simulink model "structuri_avansate"  (R2024a)
settings: Solver=VariableStepAuto  StartTime=0.0  StopTime=1000  RelTol=1e-3
values from neighbouring files (symbols this model uses):
  C = 9    [Proiect.m]
  h0 = 16.78    [Proiect.m]
  h1 = 19.66    [Proiect.m]
  k = 0.035    [Proiect.m]
  k11 = k2*k2+4*(k-k3)*k1    (= 0.0890826)    [Proiect.m]
  k12 = 8*(k-k3)    (= 0.2848)    [Proiect.m]
  k13 = 2*(k-k3)    (= 0.0712)    [Proiect.m]
  k2 = -0.015    [Proiect.m]
  kcompensare = (delta_h/(q1-q0))/(delta_h/delta_ua)    (= 0.16393442623)    [Proiect.m]
  kp = (delta_h/3)/delta_ua    (= 1.92)    [Proiect.m]
  q0 = 37.07    [Proiect.m]
undefined symbols (not defined in the file or in its folder): ki, ki1, ki2, kp1, kp2
libraries: slpidlib x6
(part 1 of 2)
settings Model: Creator=cernu  LastModifiedBy=cernu

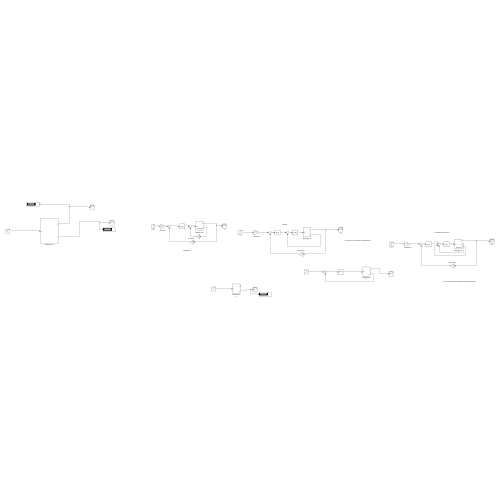
[thumbnail: Simulink's stored preview of the top-level diagram]
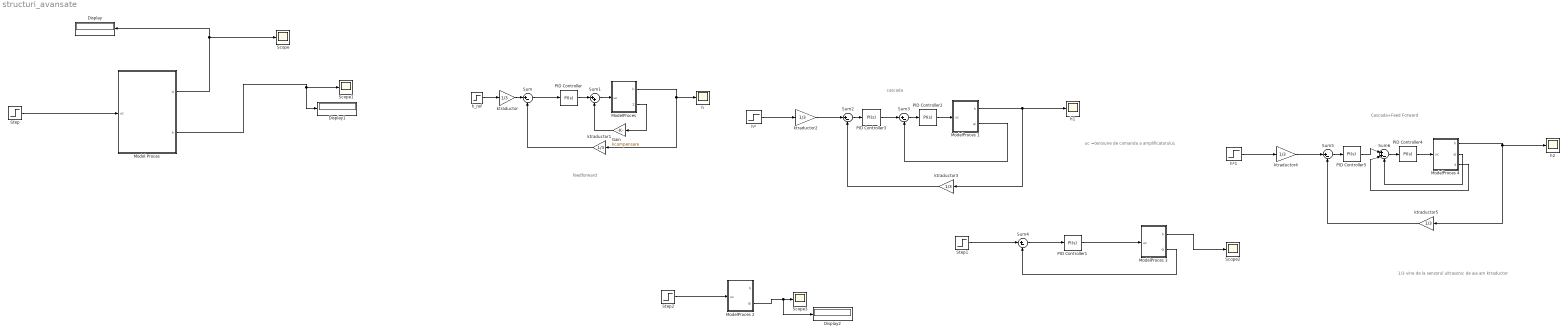
== system structuri_avansate ==
  note: 1/3 vine de la senzorul ultrasonic de aia am ktraductor
  note: Cascada+Feed Forward
  note: uc =tensiune de comanda a amplificatorului;
  note: cascada
  note: feedforward
  Display : Display
  Display1 : Display
  Display2 : Display
  Gain : Gain  Gain=kcompensare
  Model Proces : Subsystem
  "ModelProces " : Subsystem
  ModelProces 1 : Subsystem
  ModelProces 2 : Subsystem
  ModelProces 3 : Subsystem
  ModelProces 4 : Subsystem
  PID Controller : slpidlib/PID Controller  Controller=PI  Form=Parallel  TimeDomain=Continuous-time  UseExternalTs=off  SampleTime=-1  IntegratorMethod=Forward Euler  FilterMethod=Forward Euler  ControllerParametersSource=internal  P=kp  I=ki  UseKiTs=off  D=0  UseExternalDerivativeSource=off  N=100  UseFilter=on  TunerSelectOption=Transfer Function Based (PID Tuner App)  InitialConditionSource=internal  InitialConditionForIntegrator=6.7  InitialConditionForFilter=0  DifferentiatorICPrevScaledInput=0  ExternalReset=none  TrackingMode=off  Kt=1  LimitOutput=off  SatLimitsSource=internal  UpperSaturationLimit=inf  LowerSaturationLimit=-inf  LinearizeAsGain=on  AntiWindupMode=none  Kb=1  LimitIntegrator=off  UpperIntegratorSaturationLimit=inf  LowerIntegratorSaturationLimit=-inf  POutMin=[]  POutMax=[]  IOutMin=[]  IOutMax=[]  DOutMin=[]  DOutMax=[]  NOutMin=[]  NOutMax=[]  SumOutMin=[]  SumOutMax=[]  SaturationOutMin=[]  SaturationOutMax=[]  PParamMin=[]  PParamMax=[]  IParamMin=[]  IParamMax=[]  DParamMin=[]  DParamMax=[]  NParamMin=[]  NParamMax=[]  KbParamMin=[]  KbParamMax=[]  KtParamMin=[]  KtParamMax=[]  KbOutMin=[]  KbOutMax=[]  KtOutMin=[]  KtOutMax=[]  IntegratorOutMin=[]  IntegratorOutMax=[]  FilterOutMin=[]  FilterOutMax=[]  SumI1OutMin=[]  SumI1OutMax=[]  SumI2OutMin=[]  SumI2OutMax=[]  SumI3OutMin=[]  SumI3OutMax=[]  SumI4OutMin=[]  SumI4OutMax=[]  SumDOutMin=[]  SumDOutMax=[]  DifferentiatorOutMin=[]  DifferentiatorOutMax=[]  FilterDiffOutCoefMin=[]  FilterDiffOutCoefMax=[]  ReciprocalOutMin=[]  ReciprocalOutMax=[]  SumDenOutMin=[]  SumDenOutMax=[]  SumNumOutMin=[]  SumNumOutMax=[]  DivideOutMin=[]  DivideOutMax=[]  UdiffTsProdOutMin=[]  UdiffTsProdOutMax=[]  NTsProdOutMin=[]  NTsProdOutMax=[]  UintegralTsProdOutMin=[]  UintegralTsProdOutMax=[]  UngainTsProdOutMin=[]  UngainTsProdOutMax=[]  ClampingZeroOutDataTypeStr=Inherit: Inherit via back propagation  ClampingZeroOutMin=[]  ClampingZeroOutMax=[]  FilterDenConstantOutDataTypeStr=Inherit: Inherit via back propagation  FilterDenConstantOutMin=[]  FilterDenConstantOutMax=[]  PCopyOutDataTypeStr=Inherit: Inherit via back propagation  PCopyOutMin=[]  PCopyOutMax=[]  NCopyOutDataTypeStr=Inherit: Inherit via back propagation  NCopyOutMin=[]  NCopyOutMax=[]  IntegratorContinuousStateAttributes=''  IntegratorStateMustResolveToSignalObject=off  IntegratorRTWStateStorageClass=Auto  FilterContinuousStateAttributes=''  FilterStateMustResolveToSignalObject=off  FilterRTWStateStorageClass=Auto  ParallelPVariant=InternalParameters  IdealPVariant=Disabled  IVariant=InternalParameters  DVariant=Disabled  IntegratorVariant=Continuous  SatVariant=Disabled  AWVariant=Passthrough  PCopyVariant=Disabled  TRVariant=Disabled  FdbkBlocksVariant=Forward  IdealPFdbkVariant=Disabled  SatFdbkVariant=Disabled  DerivativeFilterVariant=Disabled  NVariant=Disabled  NCopyVariant=Disabled_SignalSpec  FilterICVariant=Disabled  IntegratorICVariant=InternalICs  ExternalResetVariant=Disabled  TRSumVariant=Passthrough  SumFdbkVariant=Disabled  SumVariant=Sum_PI  TsampFilterVariant=InternalTs  TsampNgainVariant=Passthrough  TsampIntegralVariant=Disabled_SignalSpec  ExternalSaturationOutDataTypeStr=Inherit: Same as second input  DerivativeSourceVariant=Disabled
  PID Controller1 : slpidlib/PID Controller  Controller=PI  Form=Parallel  TimeDomain=Continuous-time  UseExternalTs=off  SampleTime=-1  IntegratorMethod=Forward Euler  FilterMethod=Forward Euler  ControllerParametersSource=internal  P=kp1  I=ki1  UseKiTs=off  D=0  UseExternalDerivativeSource=off  N=100  UseFilter=on  TunerSelectOption=Transfer Function Based (PID Tuner App)  InitialConditionSource=internal  InitialConditionForIntegrator=6.7  InitialConditionForFilter=0  DifferentiatorICPrevScaledInput=0  ExternalReset=none  TrackingMode=off  Kt=1  LimitOutput=off  SatLimitsSource=internal  UpperSaturationLimit=inf  LowerSaturationLimit=-inf  LinearizeAsGain=on  AntiWindupMode=none  Kb=1  LimitIntegrator=off  UpperIntegratorSaturationLimit=inf  LowerIntegratorSaturationLimit=-inf  POutMin=[]  POutMax=[]  IOutMin=[]  IOutMax=[]  DOutMin=[]  DOutMax=[]  NOutMin=[]  NOutMax=[]  SumOutMin=[]  SumOutMax=[]  SaturationOutMin=[]  SaturationOutMax=[]  PParamMin=[]  PParamMax=[]  IParamMin=[]  IParamMax=[]  DParamMin=[]  DParamMax=[]  NParamMin=[]  NParamMax=[]  KbParamMin=[]  KbParamMax=[]  KtParamMin=[]  KtParamMax=[]  KbOutMin=[]  KbOutMax=[]  KtOutMin=[]  KtOutMax=[]  IntegratorOutMin=[]  IntegratorOutMax=[]  FilterOutMin=[]  FilterOutMax=[]  SumI1OutMin=[]  SumI1OutMax=[]  SumI2OutMin=[]  SumI2OutMax=[]  SumI3OutMin=[]  SumI3OutMax=[]  SumI4OutMin=[]  SumI4OutMax=[]  SumDOutMin=[]  SumDOutMax=[]  DifferentiatorOutMin=[]  DifferentiatorOutMax=[]  FilterDiffOutCoefMin=[]  FilterDiffOutCoefMax=[]  ReciprocalOutMin=[]  ReciprocalOutMax=[]  SumDenOutMin=[]  SumDenOutMax=[]  SumNumOutMin=[]  SumNumOutMax=[]  DivideOutMin=[]  DivideOutMax=[]  UdiffTsProdOutMin=[]  UdiffTsProdOutMax=[]  NTsProdOutMin=[]  NTsProdOutMax=[]  UintegralTsProdOutMin=[]  UintegralTsProdOutMax=[]  UngainTsProdOutMin=[]  UngainTsProdOutMax=[]  ClampingZeroOutDataTypeStr=Inherit: Inherit via back propagation  ClampingZeroOutMin=[]  ClampingZeroOutMax=[]  FilterDenConstantOutDataTypeStr=Inherit: Inherit via back propagation  FilterDenConstantOutMin=[]  FilterDenConstantOutMax=[]  PCopyOutDataTypeStr=Inherit: Inherit via back propagation  PCopyOutMin=[]  PCopyOutMax=[]  NCopyOutDataTypeStr=Inherit: Inherit via back propagation  NCopyOutMin=[]  NCopyOutMax=[]  IntegratorContinuousStateAttributes=''  IntegratorStateMustResolveToSignalObject=off  IntegratorRTWStateStorageClass=Auto  FilterContinuousStateAttributes=''  FilterStateMustResolveToSignalObject=off  FilterRTWStateStorageClass=Auto  ParallelPVariant=InternalParameters  IdealPVariant=Disabled  IVariant=InternalParameters  DVariant=Disabled  IntegratorVariant=Continuous  SatVariant=Disabled  AWVariant=Passthrough  PCopyVariant=Disabled  TRVariant=Disabled  FdbkBlocksVariant=Forward  IdealPFdbkVariant=Disabled  SatFdbkVariant=Disabled  DerivativeFilterVariant=Disabled  NVariant=Disabled  NCopyVariant=Disabled_SignalSpec  FilterICVariant=Disabled  IntegratorICVariant=InternalICs  ExternalResetVariant=Disabled  TRSumVariant=Passthrough  SumFdbkVariant=Disabled  SumVariant=Sum_PI  TsampFilterVariant=InternalTs  TsampNgainVariant=Passthrough  TsampIntegralVariant=Disabled_SignalSpec  ExternalSaturationOutDataTypeStr=Inherit: Same as second input  DerivativeSourceVariant=Disabled
  PID Controller2 : slpidlib/PID Controller  Controller=PI  Form=Parallel  TimeDomain=Continuous-time  UseExternalTs=off  SampleTime=-1  IntegratorMethod=Forward Euler  FilterMethod=Forward Euler  ControllerParametersSource=internal  P=kp1  I=ki1  UseKiTs=off  D=0  UseExternalDerivativeSource=off  N=100  UseFilter=on  TunerSelectOption=Transfer Function Based (PID Tuner App)  InitialConditionSource=internal  InitialConditionForIntegrator=6.7  InitialConditionForFilter=0  DifferentiatorICPrevScaledInput=0  ExternalReset=none  TrackingMode=off  Kt=1  LimitOutput=off  SatLimitsSource=internal  UpperSaturationLimit=inf  LowerSaturationLimit=-inf  LinearizeAsGain=on  AntiWindupMode=none  Kb=1  LimitIntegrator=off  UpperIntegratorSaturationLimit=inf  LowerIntegratorSaturationLimit=-inf  POutMin=[]  POutMax=[]  IOutMin=[]  IOutMax=[]  DOutMin=[]  DOutMax=[]  NOutMin=[]  NOutMax=[]  SumOutMin=[]  SumOutMax=[]  SaturationOutMin=[]  SaturationOutMax=[]  PParamMin=[]  PParamMax=[]  IParamMin=[]  IParamMax=[]  DParamMin=[]  DParamMax=[]  NParamMin=[]  NParamMax=[]  KbParamMin=[]  KbParamMax=[]  KtParamMin=[]  KtParamMax=[]  KbOutMin=[]  KbOutMax=[]  KtOutMin=[]  KtOutMax=[]  IntegratorOutMin=[]  IntegratorOutMax=[]  FilterOutMin=[]  FilterOutMax=[]  SumI1OutMin=[]  SumI1OutMax=[]  SumI2OutMin=[]  SumI2OutMax=[]  SumI3OutMin=[]  SumI3OutMax=[]  SumI4OutMin=[]  SumI4OutMax=[]  SumDOutMin=[]  SumDOutMax=[]  DifferentiatorOutMin=[]  DifferentiatorOutMax=[]  FilterDiffOutCoefMin=[]  FilterDiffOutCoefMax=[]  ReciprocalOutMin=[]  ReciprocalOutMax=[]  SumDenOutMin=[]  SumDenOutMax=[]  SumNumOutMin=[]  SumNumOutMax=[]  DivideOutMin=[]  DivideOutMax=[]  UdiffTsProdOutMin=[]  UdiffTsProdOutMax=[]  NTsProdOutMin=[]  NTsProdOutMax=[]  UintegralTsProdOutMin=[]  UintegralTsProdOutMax=[]  UngainTsProdOutMin=[]  UngainTsProdOutMax=[]  ClampingZeroOutDataTypeStr=Inherit: Inherit via back propagation  ClampingZeroOutMin=[]  ClampingZeroOutMax=[]  FilterDenConstantOutDataTypeStr=Inherit: Inherit via back propagation  FilterDenConstantOutMin=[]  FilterDenConstantOutMax=[]  PCopyOutDataTypeStr=Inherit: Inherit via back propagation  PCopyOutMin=[]  PCopyOutMax=[]  NCopyOutDataTypeStr=Inherit: Inherit via back propagation  NCopyOutMin=[]  NCopyOutMax=[]  IntegratorContinuousStateAttributes=''  IntegratorStateMustResolveToSignalObject=off  IntegratorRTWStateStorageClass=Auto  FilterContinuousStateAttributes=''  FilterStateMustResolveToSignalObject=off  FilterRTWStateStorageClass=Auto  ParallelPVariant=InternalParameters  IdealPVariant=Disabled  IVariant=InternalParameters  DVariant=Disabled  IntegratorVariant=Continuous  SatVariant=Disabled  AWVariant=Passthrough  PCopyVariant=Disabled  TRVariant=Disabled  FdbkBlocksVariant=Forward  IdealPFdbkVariant=Disabled  SatFdbkVariant=Disabled  DerivativeFilterVariant=Disabled  NVariant=Disabled  NCopyVariant=Disabled_SignalSpec  FilterICVariant=Disabled  IntegratorICVariant=InternalICs  ExternalResetVariant=Disabled  TRSumVariant=Passthrough  SumFdbkVariant=Disabled  SumVariant=Sum_PI  TsampFilterVariant=InternalTs  TsampNgainVariant=Passthrough  TsampIntegralVariant=Disabled_SignalSpec  ExternalSaturationOutDataTypeStr=Inherit: Same as second input  DerivativeSourceVariant=Disabled
  PID Controller3 : slpidlib/PID Controller  Controller=PI  Form=Parallel  TimeDomain=Continuous-time  UseExternalTs=off  SampleTime=-1  IntegratorMethod=Forward Euler  FilterMethod=Forward Euler  ControllerParametersSource=internal  P=kp2  I=ki2  UseKiTs=off  D=0  UseExternalDerivativeSource=off  N=100  UseFilter=on  TunerSelectOption=Transfer Function Based (PID Tuner App)  InitialConditionSource=internal  InitialConditionForIntegrator=q0  InitialConditionForFilter=0  DifferentiatorICPrevScaledInput=0  ExternalReset=none  TrackingMode=off  Kt=1  LimitOutput=off  SatLimitsSource=internal  UpperSaturationLimit=inf  LowerSaturationLimit=-inf  LinearizeAsGain=on  AntiWindupMode=none  Kb=1  LimitIntegrator=off  UpperIntegratorSaturationLimit=inf  LowerIntegratorSaturationLimit=-inf  POutMin=[]  POutMax=[]  IOutMin=[]  IOutMax=[]  DOutMin=[]  DOutMax=[]  NOutMin=[]  NOutMax=[]  SumOutMin=[]  SumOutMax=[]  SaturationOutMin=[]  SaturationOutMax=[]  PParamMin=[]  PParamMax=[]  IParamMin=[]  IParamMax=[]  DParamMin=[]  DParamMax=[]  NParamMin=[]  NParamMax=[]  KbParamMin=[]  KbParamMax=[]  KtParamMin=[]  KtParamMax=[]  KbOutMin=[]  KbOutMax=[]  KtOutMin=[]  KtOutMax=[]  IntegratorOutMin=[]  IntegratorOutMax=[]  FilterOutMin=[]  FilterOutMax=[]  SumI1OutMin=[]  SumI1OutMax=[]  SumI2OutMin=[]  SumI2OutMax=[]  SumI3OutMin=[]  SumI3OutMax=[]  SumI4OutMin=[]  SumI4OutMax=[]  SumDOutMin=[]  SumDOutMax=[]  DifferentiatorOutMin=[]  DifferentiatorOutMax=[]  FilterDiffOutCoefMin=[]  FilterDiffOutCoefMax=[]  ReciprocalOutMin=[]  ReciprocalOutMax=[]  SumDenOutMin=[]  SumDenOutMax=[]  SumNumOutMin=[]  SumNumOutMax=[]  DivideOutMin=[]  DivideOutMax=[]  UdiffTsProdOutMin=[]  UdiffTsProdOutMax=[]  NTsProdOutMin=[]  NTsProdOutMax=[]  UintegralTsProdOutMin=[]  UintegralTsProdOutMax=[]  UngainTsProdOutMin=[]  UngainTsProdOutMax=[]  ClampingZeroOutDataTypeStr=Inherit: Inherit via back propagation  ClampingZeroOutMin=[]  ClampingZeroOutMax=[]  FilterDenConstantOutDataTypeStr=Inherit: Inherit via back propagation  FilterDenConstantOutMin=[]  FilterDenConstantOutMax=[]  PCopyOutDataTypeStr=Inherit: Inherit via back propagation  PCopyOutMin=[]  PCopyOutMax=[]  NCopyOutDataTypeStr=Inherit: Inherit via back propagation  NCopyOutMin=[]  NCopyOutMax=[]  IntegratorContinuousStateAttributes=''  IntegratorStateMustResolveToSignalObject=off  IntegratorRTWStateStorageClass=Auto  FilterContinuousStateAttributes=''  FilterStateMustResolveToSignalObject=off  FilterRTWStateStorageClass=Auto  ParallelPVariant=InternalParameters  IdealPVariant=Disabled  IVariant=InternalParameters  DVariant=Disabled  IntegratorVariant=Continuous  SatVariant=Disabled  AWVariant=Passthrough  PCopyVariant=Disabled  TRVariant=Disabled  FdbkBlocksVariant=Forward  IdealPFdbkVariant=Disabled  SatFdbkVariant=Disabled  DerivativeFilterVariant=Disabled  NVariant=Disabled  NCopyVariant=Disabled_SignalSpec  FilterICVariant=Disabled  IntegratorICVariant=InternalICs  ExternalResetVariant=Disabled  TRSumVariant=Passthrough  SumFdbkVariant=Disabled  SumVariant=Sum_PI  TsampFilterVariant=InternalTs  TsampNgainVariant=Passthrough  TsampIntegralVariant=Disabled_SignalSpec  ExternalSaturationOutDataTypeStr=Inherit: Same as second input  DerivativeSourceVariant=Disabled
  PID Controller4 : slpidlib/PID Controller  Controller=PI  Form=Parallel  TimeDomain=Continuous-time  UseExternalTs=off  SampleTime=-1  IntegratorMethod=Forward Euler  FilterMethod=Forward Euler  ControllerParametersSource=internal  P=kp1  I=ki1  UseKiTs=off  D=0  UseExternalDerivativeSource=off  N=100  UseFilter=on  TunerSelectOption=Transfer Function Based (PID Tuner App)  InitialConditionSource=internal  InitialConditionForIntegrator=6.7  InitialConditionForFilter=0  DifferentiatorICPrevScaledInput=0  ExternalReset=none  TrackingMode=off  Kt=1  LimitOutput=off  SatLimitsSource=internal  UpperSaturationLimit=inf  LowerSaturationLimit=-inf  LinearizeAsGain=on  AntiWindupMode=none  Kb=1  LimitIntegrator=off  UpperIntegratorSaturationLimit=inf  LowerIntegratorSaturationLimit=-inf  POutMin=[]  POutMax=[]  IOutMin=[]  IOutMax=[]  DOutMin=[]  DOutMax=[]  NOutMin=[]  NOutMax=[]  SumOutMin=[]  SumOutMax=[]  SaturationOutMin=[]  SaturationOutMax=[]  PParamMin=[]  PParamMax=[]  IParamMin=[]  IParamMax=[]  DParamMin=[]  DParamMax=[]  NParamMin=[]  NParamMax=[]  KbParamMin=[]  KbParamMax=[]  KtParamMin=[]  KtParamMax=[]  KbOutMin=[]  KbOutMax=[]  KtOutMin=[]  KtOutMax=[]  IntegratorOutMin=[]  IntegratorOutMax=[]  FilterOutMin=[]  FilterOutMax=[]  SumI1OutMin=[]  SumI1OutMax=[]  SumI2OutMin=[]  SumI2OutMax=[]  SumI3OutMin=[]  SumI3OutMax=[]  SumI4OutMin=[]  SumI4OutMax=[]  SumDOutMin=[]  SumDOutMax=[]  DifferentiatorOutMin=[]  DifferentiatorOutMax=[]  FilterDiffOutCoefMin=[]  FilterDiffOutCoefMax=[]  ReciprocalOutMin=[]  ReciprocalOutMax=[]  SumDenOutMin=[]  SumDenOutMax=[]  SumNumOutMin=[]  SumNumOutMax=[]  DivideOutMin=[]  DivideOutMax=[]  UdiffTsProdOutMin=[]  UdiffTsProdOutMax=[]  NTsProdOutMin=[]  NTsProdOutMax=[]  UintegralTsProdOutMin=[]  UintegralTsProdOutMax=[]  UngainTsProdOutMin=[]  UngainTsProdOutMax=[]  ClampingZeroOutDataTypeStr=Inherit: Inherit via back propagation  ClampingZeroOutMin=[]  ClampingZeroOutMax=[]  FilterDenConstantOutDataTypeStr=Inherit: Inherit via back propagation  FilterDenConstantOutMin=[]  FilterDenConstantOutMax=[]  PCopyOutDataTypeStr=Inherit: Inherit via back propagation  PCopyOutMin=[]  PCopyOutMax=[]  NCopyOutDataTypeStr=Inherit: Inherit via back propagation  NCopyOutMin=[]  NCopyOutMax=[]  IntegratorContinuousStateAttributes=''  IntegratorStateMustResolveToSignalObject=off  IntegratorRTWStateStorageClass=Auto  FilterContinuousStateAttributes=''  FilterStateMustResolveToSignalObject=off  FilterRTWStateStorageClass=Auto  ParallelPVariant=InternalParameters  IdealPVariant=Disabled  IVariant=InternalParameters  DVariant=Disabled  IntegratorVariant=Continuous  SatVariant=Disabled  AWVariant=Passthrough  PCopyVariant=Disabled  TRVariant=Disabled  FdbkBlocksVariant=Forward  IdealPFdbkVariant=Disabled  SatFdbkVariant=Disabled  DerivativeFilterVariant=Disabled  NVariant=Disabled  NCopyVariant=Disabled_SignalSpec  FilterICVariant=Disabled  IntegratorICVariant=InternalICs  ExternalResetVariant=Disabled  TRSumVariant=Passthrough  SumFdbkVariant=Disabled  SumVariant=Sum_PI  TsampFilterVariant=InternalTs  TsampNgainVariant=Passthrough  TsampIntegralVariant=Disabled_SignalSpec  ExternalSaturationOutDataTypeStr=Inherit: Same as second input  DerivativeSourceVariant=Disabled
  PID Controller5 : slpidlib/PID Controller  Controller=PI  Form=Parallel  TimeDomain=Continuous-time  UseExternalTs=off  SampleTime=-1  IntegratorMethod=Forward Euler  FilterMethod=Forward Euler  ControllerParametersSource=internal  P=kp2  I=ki2  UseKiTs=off  D=0  UseExternalDerivativeSource=off  N=100  UseFilter=on  TunerSelectOption=Transfer Function Based (PID Tuner App)  InitialConditionSource=internal  InitialConditionForIntegrator=q0  InitialConditionForFilter=0  DifferentiatorICPrevScaledInput=0  ExternalReset=none  TrackingMode=off  Kt=1  LimitOutput=off  SatLimitsSource=internal  UpperSaturationLimit=inf  LowerSaturationLimit=-inf  LinearizeAsGain=on  AntiWindupMode=none  Kb=1  LimitIntegrator=off  UpperIntegratorSaturationLimit=inf  LowerIntegratorSaturationLimit=-inf  POutMin=[]  POutMax=[]  IOutMin=[]  IOutMax=[]  DOutMin=[]  DOutMax=[]  NOutMin=[]  NOutMax=[]  SumOutMin=[]  SumOutMax=[]  SaturationOutMin=[]  SaturationOutMax=[]  PParamMin=[]  PParamMax=[]  IParamMin=[]  IParamMax=[]  DParamMin=[]  DParamMax=[]  NParamMin=[]  NParamMax=[]  KbParamMin=[]  KbParamMax=[]  KtParamMin=[]  KtParamMax=[]  KbOutMin=[]  KbOutMax=[]  KtOutMin=[]  KtOutMax=[]  IntegratorOutMin=[]  IntegratorOutMax=[]  FilterOutMin=[]  FilterOutMax=[]  SumI1OutMin=[]  SumI1OutMax=[]  SumI2OutMin=[]  SumI2OutMax=[]  SumI3OutMin=[]  SumI3OutMax=[]  SumI4OutMin=[]  SumI4OutMax=[]  SumDOutMin=[]  SumDOutMax=[]  DifferentiatorOutMin=[]  DifferentiatorOutMax=[]  FilterDiffOutCoefMin=[]  FilterDiffOutCoefMax=[]  ReciprocalOutMin=[]  ReciprocalOutMax=[]  SumDenOutMin=[]  SumDenOutMax=[]  SumNumOutMin=[]  SumNumOutMax=[]  DivideOutMin=[]  DivideOutMax=[]  UdiffTsProdOutMin=[]  UdiffTsProdOutMax=[]  NTsProdOutMin=[]  NTsProdOutMax=[]  UintegralTsProdOutMin=[]  UintegralTsProdOutMax=[]  UngainTsProdOutMin=[]  UngainTsProdOutMax=[]  ClampingZeroOutDataTypeStr=Inherit: Inherit via back propagation  ClampingZeroOutMin=[]  ClampingZeroOutMax=[]  FilterDenConstantOutDataTypeStr=Inherit: Inherit via back propagation  FilterDenConstantOutMin=[]  FilterDenConstantOutMax=[]  PCopyOutDataTypeStr=Inherit: Inherit via back propagation  PCopyOutMin=[]  PCopyOutMax=[]  NCopyOutDataTypeStr=Inherit: Inherit via back propagation  NCopyOutMin=[]  NCopyOutMax=[]  IntegratorContinuousStateAttributes=''  IntegratorStateMustResolveToSignalObject=off  IntegratorRTWStateStorageClass=Auto  FilterContinuousStateAttributes=''  FilterStateMustResolveToSignalObject=off  FilterRTWStateStorageClass=Auto  ParallelPVariant=InternalParameters  IdealPVariant=Disabled  IVariant=InternalParameters  DVariant=Disabled  IntegratorVariant=Continuous  SatVariant=Disabled  AWVariant=Passthrough  PCopyVariant=Disabled  TRVariant=Disabled  FdbkBlocksVariant=Forward  IdealPFdbkVariant=Disabled  SatFdbkVariant=Disabled  DerivativeFilterVariant=Disabled  NVariant=Disabled  NCopyVariant=Disabled_SignalSpec  FilterICVariant=Disabled  IntegratorICVariant=InternalICs  ExternalResetVariant=Disabled  TRSumVariant=Passthrough  SumFdbkVariant=Disabled  SumVariant=Sum_PI  TsampFilterVariant=InternalTs  TsampNgainVariant=Passthrough  TsampIntegralVariant=Disabled_SignalSpec  ExternalSaturationOutDataTypeStr=Inherit: Same as second input  DerivativeSourceVariant=Disabled
  Scope{,1..3} (4 alike) : Scope
  Step : Step  Time=0  Before=6.7  After=7.2  SampleTime=0
  Step1 : Step  Time=0  Before=q0  After=46.21  SampleTime=0
  Step2 : Step  Time=0  Before=6.7  After=7.2  SampleTime=0
  Sum{,2..5} (5 alike) : Sum  Inputs=|+-
  Sum1 : Sum  Inputs=|++
  Sum6 : Sum  Inputs=|++-
  h : Scope
  h* : Step  Time=0  Before=h0  After=h1  SampleTime=0
  h*1 : Step  Time=0  Before=h0  After=h1  SampleTime=0
  h1 : Scope
  h2 : Scope
  h_ref : Step  Time=0  Before=h0  After=h1  SampleTime=0
  ktraductor{,1..5} (6 alike) : Gain  Gain=1/3
  wires:
  Model Proces/1(q) -> Display/1, Scope/1
  Model Proces/2(h) -> Scope1/1, Display1/1
  Step/1 -> Model Proces/1(uc)
  "ModelProces "/2(perturbatie) -> Gain/1
  Sum1/1 -> "ModelProces "/1(uc)
  ktraductor1/1 -> Sum/2
  PID Controller/1 -> Sum1/1
  ktraductor/1 -> Sum/1
  Gain/1 -> Sum1/2
  "ModelProces "/1(h) -> h/1, ktraductor1/1
  h_ref/1 -> ktraductor/1
  Sum/1 -> PID Controller/1
  h*/1 -> ktraductor2/1
  Sum2/1 -> PID Controller3/1
  PID Controller2/1 -> ModelProces 1/1(uc)
  ModelProces 1/2(qi) -> Sum3/2
  ModelProces 1/1(h) -> ktraductor3/1, h1/1
  ktraductor3/1 -> Sum2/2
  ktraductor2/1 -> Sum2/1
  PID Controller3/1 -> Sum3/1
  Sum3/1 -> PID Controller2/1
  Step2/1 -> ModelProces 2/1(uc)
  ModelProces 2/2(qi) -> Display2/1, Scope3/1
  Sum4/1 -> PID Controller1/1
  PID Controller1/1 -> ModelProces 3/1(uc)
  Step1/1 -> Sum4/1
  ModelProces 3/1(h) -> Scope2/1
  ModelProces 3/2(qi) -> Sum4/2
  PID Controller5/1 -> Sum6/1
  Sum5/1 -> PID Controller5/1
  ktraductor5/1 -> Sum5/2
  Sum6/1 -> PID Controller4/1
  PID Controller4/1 -> ModelProces 4/1(uc)
  h*1/1 -> ktraductor4/1
  ModelProces 4/1(h) -> ktraductor5/1, h2/1
  ktraductor4/1 -> Sum5/1
  ModelProces 4/3(Peturbatie) -> Sum6/2
  ModelProces 4/2(qi) -> Sum6/3

== system structuri_avansate/Model Proces ==
  uc : Inport
  Amplificator : Subsystem
  Curent robotic : Subsystem
  Filtru : Subsystem
  Motor : Subsystem
  Pompa : Subsystem
  Randament pompa : Subsystem
  Rezervor : Subsystem
  q : Outport
  h : Outport  Port=2
  wires:
  Curent robotic/1(im) -> Motor/2(im)
  Rezervor/1(h) -> h/1, Curent robotic/1(h), Pompa/2(h)
  Amplificator/1(um) -> Curent robotic/4(um), Randament pompa/2(um), Motor/1(um)
  Filtru/1(q2) -> q/1, Curent robotic/2(q), Randament pompa/1(q), Rezervor/1(ln1)
  Randament pompa/1(eta) -> Curent robotic/3(eta)
  uc/1 -> Amplificator/1(ua)
  Motor/1(kn) -> Pompa/1(kn)
  Pompa/1(q) -> Filtru/1(q1)

== system structuri_avansate/ModelProces  ==
  uc : Inport
  "Amplificator " : Subsystem
  Curentul_rotoric : Subsystem
  Filtru : Subsystem
  "Motor " : Subsystem
  Pompa : Subsystem
  Randament : Subsystem
  Rezervor : Subsystem
  h : Outport
  perturbatie : Outport  Port=2
  wires:
  "Amplificator "/1("um ") -> "Motor "/1(um), Randament/2(um), Curentul_rotoric/4(um)
  "Motor "/1(kn) -> Pompa/1(kn)
  Pompa/1(q) -> Filtru/1(q)
  Filtru/1(q_f) -> Randament/1("q "), Curentul_rotoric/1(q), Rezervor/1(q)
  Rezervor/1(h) -> h/1, Curentul_rotoric/3(h), Pompa/2(h)
  Curentul_rotoric/1(im) -> "Motor "/2(im)
  Randament/1("eta ") -> Curentul_rotoric/2(eta)
  uc/1 -> "Amplificator "/1(ua)
  Rezervor/2(perturbatie) -> perturbatie/1

== system structuri_avansate/ModelProces 1 ==
  uc : Inport
  "Amplificator " : Subsystem
  Curentul_rotoric : Subsystem
  Filtru : Subsystem
  "Motor " : Subsystem
  Pompa : Subsystem
  Randament : Subsystem
  Rezervor : Subsystem
  perturbatie k : Step  Time=300  After=0.09  SampleTime=0
  h : Outport
  qi : Outport  Port=2
  wires:
  "Amplificator "/1("um ") -> "Motor "/1(um), Randament/2(um), Curentul_rotoric/4(um)
  Filtru/1(q_f) -> Rezervor/1(q), qi/1, Randament/1("q "), Curentul_rotoric/1(q)
  Rezervor/1(h) -> h/1, Curentul_rotoric/3(h), Pompa/1(h)
  Curentul_rotoric/1(im) -> "Motor "/2(im)
  Randament/1("eta ") -> Curentul_rotoric/2(eta)
  uc/1 -> "Amplificator "/1(ua)
  Pompa/1(q) -> Filtru/1(q)
  perturbatie k/1 -> Pompa/2(perturbatie k)
  "Motor "/1(kn) -> Pompa/3(kn)

== system structuri_avansate/ModelProces 2 ==
  uc : Inport
  "Amplificator " : Subsystem
  Curentul_rotoric : Subsystem
  Filtru : Subsystem
  "Motor " : Subsystem
  Pompa : Subsystem
  Randament : Subsystem
  Rezervor : Subsystem
  perturbatie k : Step  Time=300  After=0.03  SampleTime=0
  h : Outport
  qi : Outport  Port=2
  wires:
  "Amplificator "/1("um ") -> "Motor "/1(um), Randament/2(um), Curentul_rotoric/4(um)
  Filtru/1(q_f) -> Rezervor/1(q), qi/1, Randament/1("q "), Curentul_rotoric/1(q)
  Rezervor/1(h) -> h/1, Curentul_rotoric/3(h), Pompa/1(h)
  Curentul_rotoric/1(im) -> "Motor "/2(im)
  Randament/1("eta ") -> Curentul_rotoric/2(eta)
  uc/1 -> "Amplificator "/1(ua)
  Pompa/1(q) -> Filtru/1(q)
  perturbatie k/1 -> Pompa/2(perturbatie k)
  "Motor "/1(kn) -> Pompa/3(kn)

== system structuri_avansate/ModelProces 3 ==
  uc : Inport
  "Amplificator " : Subsystem
  Curentul_rotoric : Subsystem
  Filtru : Subsystem
  "Motor " : Subsystem
  Pompa : Subsystem
  Randament : Subsystem
  Rezervor : Subsystem
  perturbatie k : Step  Time=300  After=0.03  SampleTime=0
  h : Outport
  qi : Outport  Port=2
  wires:
  "Amplificator "/1("um ") -> "Motor "/1(um), Randament/2(um), Curentul_rotoric/4(um)
  Filtru/1(q_f) -> Rezervor/1(q), qi/1, Randament/1("q "), Curentul_rotoric/1(q)
  Rezervor/1(h) -> h/1, Curentul_rotoric/3(h), Pompa/1(h)
  Curentul_rotoric/1(im) -> "Motor "/2(im)
  Randament/1("eta ") -> Curentul_rotoric/2(eta)
  uc/1 -> "Amplificator "/1(ua)
  Pompa/1(q) -> Filtru/1(q)
  perturbatie k/1 -> Pompa/2(perturbatie k)
  "Motor "/1(kn) -> Pompa/3(kn)

== system structuri_avansate/ModelProces 4 ==
  uc : Inport
  "Amplificator " : Subsystem
  Curentul_rotoric : Subsystem
  Filtru : Subsystem
  "Motor " : Subsystem
  Pompa : Subsystem
  Randament : Subsystem
  Rezervor : Subsystem
  perturbatie k : Step  Time=300  After=-0.04  SampleTime=0
  h : Outport
  qi : Outport  Port=2
  Peturbatie : Outport  Port=3
  wires:
  "Amplificator "/1("um ") -> "Motor "/1(um), Randament/2(um), Curentul_rotoric/4(um)
  Filtru/1(q_f) -> Rezervor/1(q), qi/1, Randament/1("q "), Curentul_rotoric/1(q)
  Rezervor/1(h) -> h/1, Curentul_rotoric/3(h), Pompa/1(h)
  Curentul_rotoric/1(im) -> "Motor "/2(im)
  Randament/1("eta ") -> Curentul_rotoric/2(eta)
  uc/1 -> "Amplificator "/1(ua)
  Pompa/1(q) -> Filtru/1(q)
  perturbatie k/1 -> Pompa/2(perturbatie k)
  "Motor "/1(kn) -> Pompa/3(kn)
  Rezervor/2(perturbatie) -> Peturbatie/1

== system structuri_avansate/Model Proces/Amplificator ==
  ua : Inport
  Constant : Constant  Value=8.1
  Gain : Gain  Gain=2.2
  Gain1 : Gain  Gain=2.2
  Gain2 : Gain  Gain=5
  Saturation : Saturate  UpperLimit=22  LowerLimit=0
  Sum : Sum  Inputs=|+-
  Sum1 : Sum  Inputs=|++
  Switch : Switch  Criteria=u2 > Threshold  Threshold=8.1  SaturateOnIntegerOverflow=off  InputSameDT=off
  um : Outport
  wires:
  Saturation/1 -> um/1
  Sum/1 -> Gain2/1
  Constant/1 -> Sum/2
  Sum1/1 -> Switch/1
  Gain1/1 -> Sum1/1
  ua/1 -> Sum/1, Gain1/1, Switch/2, Gain/1
  Gain2/1 -> Sum1/2
  Switch/1 -> Saturation/1
  Gain/1 -> Switch/3

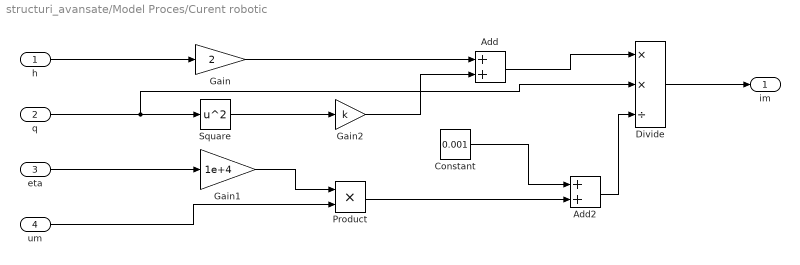
== system structuri_avansate/Model Proces/Curent robotic ==
  h : Inport
  q : Inport  Port=2
  eta : Inport  Port=3
  um : Inport  Port=4
  Add : Sum
  Add2 : Sum
  Constant : Constant  Value=0.001
  Divide : Product  Inputs=**/
  Gain : Gain  Gain=2
  Gain1 : Gain  Gain=1e+4
  Gain2 : Gain  Gain=k
  Product : Product
  Square : Math  Operator=square
  im : Outport
  wires:
  Gain2/1 -> Add/2
  Gain1/1 -> Product/1
  q/1 -> Divide/2, Square/1
  Divide/1 -> im/1
  h/1 -> Gain/1
  Add/1 -> Divide/1
  Constant/1 -> Add2/1
  um/1 -> Product/2
  Gain/1 -> Add/1
  Product/1 -> Add2/2
  Square/1 -> Gain2/1
  eta/1 -> Gain1/1
  Add2/1 -> Divide/3

== system structuri_avansate/Model Proces/Filtru ==
  q1 : Inport
  Integrator : Integrator  InitialCondition=q0
  Sum : Sum  Inputs=|+-
  q2 : Outport
  wires:
  Integrator/1 -> q2/1, Sum/2
  Sum/1 -> Integrator/1
  q1/1 -> Sum/1

== system structuri_avansate/Model Proces/Motor ==
  um : Inport
  im : Inport  Port=2
  Add : Sum  Inputs=+-
  Rm : Gain  Gain=3
  kn : Outport
  wires:
  um/1 -> Add/1
  im/1 -> Rm/1
  Rm/1 -> Add/2
  Add/1 -> kn/1

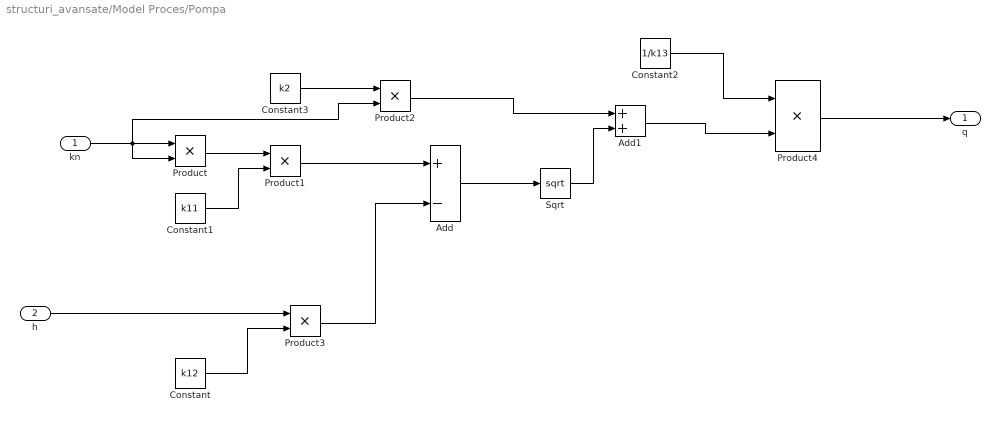
== system structuri_avansate/Model Proces/Pompa ==
  kn : Inport
  h : Inport  Port=2
  Add : Sum  Inputs=+-
  Add1 : Sum
  Constant : Constant  Value=k12
  Constant1 : Constant  Value=k11
  Constant2 : Constant  Value=1/k13
  Constant3 : Constant  Value=k2
  Product{,1..4} (5 alike) : Product
  Sqrt : Sqrt
  q : Outport
  wires:
  Constant2/1 -> Product4/1
  h/1 -> Product3/1
  Product4/1 -> q/1
  kn/1 -> Product2/2, Product/2, Product/1
  Constant1/1 -> Product1/2
  Constant3/1 -> Product2/1
  Product/1 -> Product1/1
  Product1/1 -> Add/1
  Constant/1 -> Product3/2
  Product3/1 -> Add/2
  Add/1 -> Sqrt/1
  Sqrt/1 -> Add1/2
  Product2/1 -> Add1/1
  Add1/1 -> Product4/2

== system structuri_avansate/Model Proces/Randament pompa ==
  q : Inport
  um : Inport  Port=2
  Gain : Gain  Gain=8e-5
  Product : Product
  eta : Outport
  wires:
  Gain/1 -> Product/2
  Product/1 -> eta/1
  um/1 -> Gain/1
  q/1 -> Product/1

== system structuri_avansate/Model Proces/Rezervor ==
  ln1 : Inport
  Gain : Gain  Gain=1/332.5
  Gain1 : Gain  Gain=C
  Integrator : Integrator  InitialCondition=h0
  Sqrt : Sqrt
  Sum : Sum  Inputs=|+-
  h : Outport
  wires:
  Gain/1 -> Integrator/1
  ln1/1 -> Sum/1
  Sum/1 -> Gain/1
  Integrator/1 -> h/1, Sqrt/1
  Sqrt/1 -> Gain1/1
  Gain1/1 -> Sum/2

== system structuri_avansate/ModelProces /Amplificator  ==
  ua : Inport
  Constant : Constant  Value=8.1
  Gain : Gain  Gain=2.2
  Gain1 : Gain  Gain=2.2
  Gain2 : Gain  Gain=5
  Saturation : Saturate  UpperLimit=22  LowerLimit=0
  Sum : Sum  Inputs=|++
  Sum1 : Sum  Inputs=|+-
  Switch : Switch  Threshold=8.1  SaturateOnIntegerOverflow=off  InputSameDT=off
  "um " : Outport
  wires:
  Sum1/1 -> Gain2/1
  ua/1 -> Switch/2, Gain/1, Sum1/1, Gain1/1
  Gain2/1 -> Sum/2
  Gain1/1 -> Sum/1
  Sum/1 -> Switch/1
  Gain/1 -> Switch/3
  Constant/1 -> Sum1/2
  Switch/1 -> Saturation/1
  Saturation/1 -> "um "/1

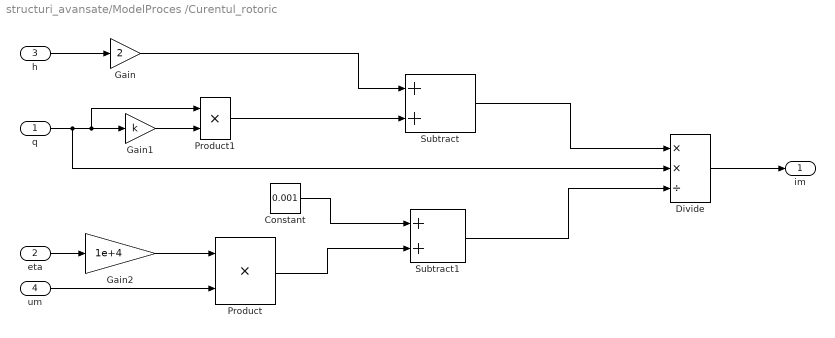
== system structuri_avansate/ModelProces /Curentul_rotoric ==
  q : Inport
  eta : Inport  Port=2
  h : Inport  Port=3
  um : Inport  Port=4
  Constant : Constant  Value=0.001
  Divide : Product  Inputs=**/
  Gain : Gain  Gain=2
  Gain1 : Gain  Gain=k
  Gain2 : Gain  Gain=1e+4
  Product : Product
  Product1 : Product
  Subtract : Sum
  Subtract1 : Sum
  im : Outport
  wires:
  h/1 -> Gain/1
  Gain/1 -> Subtract/1
  q/1 -> Divide/2, Product1/1, Gain1/1
  Gain1/1 -> Product1/2
  Product1/1 -> Subtract/2
  eta/1 -> Gain2/1
  Gain2/1 -> Product/1
  um/1 -> Product/2
  Constant/1 -> Subtract1/1
  Product/1 -> Subtract1/2
  Divide/1 -> im/1
  Subtract/1 -> Divide/1
  Subtract1/1 -> Divide/3

== system structuri_avansate/ModelProces /Filtru ==
  q : Inport
  Integrator : Integrator  InitialCondition=q0
  Sum : Sum  Inputs=|+-
  q_f : Outport
  wires:
  Integrator/1 -> Sum/2, q_f/1
  q/1 -> Sum/1
  Sum/1 -> Integrator/1

== system structuri_avansate/ModelProces /Motor  ==
  um : Inport
  im : Inport  Port=2
  Add : Sum  Inputs=+-
  Rm : Gain  Gain=3
  kn : Outport
  wires:
  Rm/1 -> Add/2
  um/1 -> Add/1
  im/1 -> Rm/1
  Add/1 -> kn/1

== system structuri_avansate/ModelProces /Pompa ==
  kn : Inport
  h : Inport  Port=2
  Gain : Gain  Gain=k2
  Gain1 : Gain  Gain=k11
  Gain2 : Gain  Gain=k12
  Gain3 : Gain  Gain=1/k13
  Product : Product
  Sqrt : Sqrt
  Subtract : Sum
  Subtract1 : Sum  Inputs=+-
  q : Outport
  wires:
  kn/1 -> Product/1, Gain/1, Product/2
  Gain3/1 -> q/1
  Subtract/1 -> Gain3/1
  Sqrt/1 -> Subtract/2
  Gain/1 -> Subtract/1
  Subtract1/1 -> Sqrt/1
  Gain1/1 -> Subtract1/1
  Gain2/1 -> Subtract1/2
  h/1 -> Gain2/1
  Product/1 -> Gain1/1

== system structuri_avansate/ModelProces /Randament ==
  "q " : Inport
  um : Inport  Port=2
  Gain : Gain  Gain=8e-5
  Product : Product
  "eta " : Outport
  wires:
  um/1 -> Gain/1
  Gain/1 -> Product/2
  "q "/1 -> Product/1
  Product/1 -> "eta "/1

== system structuri_avansate/ModelProces /Rezervor ==
  q : Inport
  Add : Sum
  Constant : Constant  Value=C
  Gain : Gain  Gain=1/332.5
  Integrator : Integrator  InitialCondition=h0
  Product : Product
  Product1 : Product
  Scope : Scope
  Sqrt : Sqrt
  Step : Step  Time=500  SampleTime=0
  Sum : Sum  Inputs=|+-
  h : Outport
  perturbatie : Outport  Port=2
  wires:
  Gain/1 -> Integrator/1
  Integrator/1 -> Sqrt/1, h/1
  q/1 -> Sum/1
  Sum/1 -> Gain/1
  Product/1 -> Scope/1, Sum/2
  Sqrt/1 -> Product1/1, Product/1
  Product1/1 -> perturbatie/1
  Step/1 -> Product1/2, Add/1
  Constant/1 -> Add/2
  Add/1 -> Product/2

== system structuri_avansate/ModelProces 1/Amplificator  ==
  ua : Inport
  Constant : Constant  Value=8.1
  Gain : Gain  Gain=2.2
  Gain1 : Gain  Gain=2.2
  Gain2 : Gain  Gain=5
  Saturation : Saturate  UpperLimit=22  LowerLimit=0
  Sum : Sum  Inputs=|++
  Sum1 : Sum  Inputs=|+-
  Switch : Switch  Threshold=8.1  SaturateOnIntegerOverflow=off  InputSameDT=off
  "um " : Outport
  wires:
  Sum1/1 -> Gain2/1
  ua/1 -> Switch/2, Gain/1, Sum1/1, Gain1/1
  Gain2/1 -> Sum/2
  Gain1/1 -> Sum/1
  Sum/1 -> Switch/1
  Gain/1 -> Switch/3
  Constant/1 -> Sum1/2
  Switch/1 -> Saturation/1
  Saturation/1 -> "um "/1

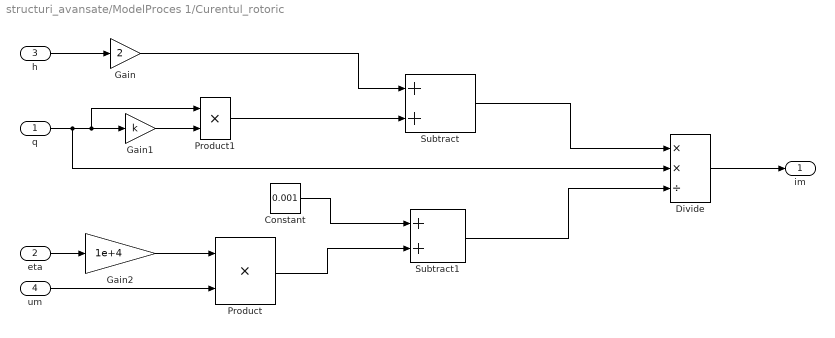
== system structuri_avansate/ModelProces 1/Curentul_rotoric ==
  q : Inport
  eta : Inport  Port=2
  h : Inport  Port=3
  um : Inport  Port=4
  Constant : Constant  Value=0.001
  Divide : Product  Inputs=**/
  Gain : Gain  Gain=2
  Gain1 : Gain  Gain=k
  Gain2 : Gain  Gain=1e+4
  Product : Product
  Product1 : Product
  Subtract : Sum
  Subtract1 : Sum
  im : Outport
  wires:
  h/1 -> Gain/1
  Gain/1 -> Subtract/1
  q/1 -> Divide/2, Product1/1, Gain1/1
  Gain1/1 -> Product1/2
  Product1/1 -> Subtract/2
  eta/1 -> Gain2/1
  Gain2/1 -> Product/1
  um/1 -> Product/2
  Constant/1 -> Subtract1/1
  Product/1 -> Subtract1/2
  Divide/1 -> im/1
  Subtract/1 -> Divide/1
  Subtract1/1 -> Divide/3

== system structuri_avansate/ModelProces 1/Filtru ==
  q : Inport
  Integrator : Integrator  InitialCondition=q0
  Sum : Sum  Inputs=|+-
  q_f : Outport
  wires:
  Integrator/1 -> Sum/2, q_f/1
  q/1 -> Sum/1
  Sum/1 -> Integrator/1

== system structuri_avansate/ModelProces 1/Motor  ==
  um : Inport
  im : Inport  Port=2
  Add : Sum  Inputs=+-
  Rm : Gain  Gain=3
  kn : Outport
  wires:
  Rm/1 -> Add/2
  um/1 -> Add/1
  im/1 -> Rm/1
  Add/1 -> kn/1

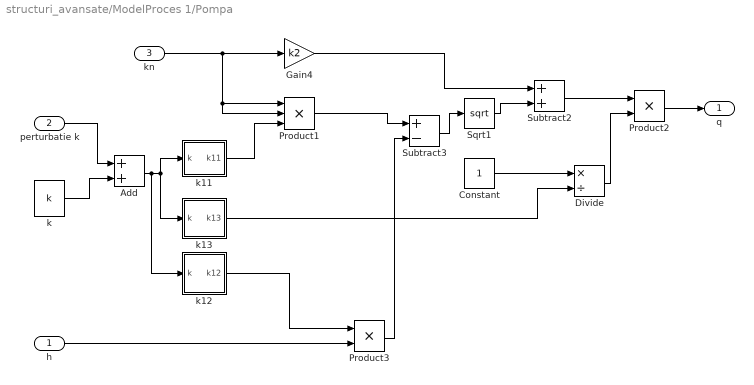
== system structuri_avansate/ModelProces 1/Pompa ==
  h : Inport
  perturbatie k : Inport  Port=2
  kn : Inport  Port=3
  Add : Sum
  Constant : Constant
  Divide : Product  Inputs=*/
  Gain4 : Gain  Gain=k2
  Product1 : Product  Inputs=3
  Product2 : Product
  Product3 : Product
  Sqrt1 : Sqrt
  Subtract2 : Sum
  Subtract3 : Sum  Inputs=+-
  "k " : Constant  Value=k
  "k11 " : Subsystem
  k12 : Subsystem
  k13 : Subsystem
  q : Outport
  wires:
  Product2/1 -> q/1
  Divide/1 -> Product2/2
  Sqrt1/1 -> Subtract2/2
  k13/1(k13) -> Divide/2
  Constant/1 -> Divide/1
  "k11 "/1(k11) -> Product1/3
  Product3/1 -> Subtract3/2
  k12/1(k12) -> Product3/1
  Subtract2/1 -> Product2/1
  Add/1 -> k12/1(k), k13/1(k), "k11 "/1(k)
  perturbatie k/1 -> Add/1
  "k "/1 -> Add/2
  Subtract3/1 -> Sqrt1/1
  kn/1 -> Product1/2, Product1/1, Gain4/1
  h/1 -> Product3/2
  Gain4/1 -> Subtract2/1
  Product1/1 -> Subtract3/1

== system structuri_avansate/ModelProces 1/Randament ==
  "q " : Inport
  um : Inport  Port=2
  Gain : Gain  Gain=8e-5
  Product : Product
  "eta " : Outport
  wires:
  um/1 -> Gain/1
  Gain/1 -> Product/2
  "q "/1 -> Product/1
  Product/1 -> "eta "/1

== system structuri_avansate/ModelProces 1/Rezervor ==
  q : Inport
  Gain : Gain  Gain=1/332.5
  Integrator : Integrator  InitialCondition=h0
  Product : Product
  Sqrt : Sqrt
  Sum : Sum  Inputs=|+-
  c : Constant  Value=C
  h : Outport
  wires:
  Sum/1 -> Gain/1
  Sqrt/1 -> Product/1
  q/1 -> Sum/1
  Gain/1 -> Integrator/1
  Product/1 -> Sum/2
  c/1 -> Product/2
  Integrator/1 -> h/1, Sqrt/1

== system structuri_avansate/ModelProces 2/Amplificator  ==
  ua : Inport
  Constant : Constant  Value=8.1
  Gain : Gain  Gain=2.2
  Gain1 : Gain  Gain=2.2
  Gain2 : Gain  Gain=5
  Saturation : Saturate  UpperLimit=22  LowerLimit=0
  Sum : Sum  Inputs=|++
  Sum1 : Sum  Inputs=|+-
  Switch : Switch  Threshold=8.1  SaturateOnIntegerOverflow=off  InputSameDT=off
  "um " : Outport
  wires:
  Sum1/1 -> Gain2/1
  ua/1 -> Switch/2, Gain/1, Sum1/1, Gain1/1
  Gain2/1 -> Sum/2
  Gain1/1 -> Sum/1
  Sum/1 -> Switch/1
  Gain/1 -> Switch/3
  Constant/1 -> Sum1/2
  Switch/1 -> Saturation/1
  Saturation/1 -> "um "/1

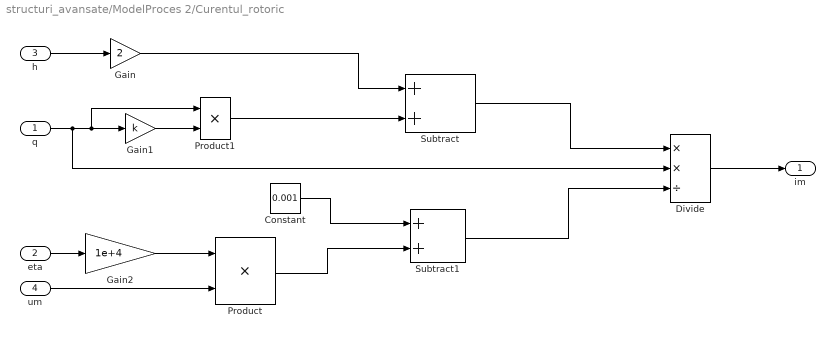
== system structuri_avansate/ModelProces 2/Curentul_rotoric ==
  q : Inport
  eta : Inport  Port=2
  h : Inport  Port=3
  um : Inport  Port=4
  Constant : Constant  Value=0.001
  Divide : Product  Inputs=**/
  Gain : Gain  Gain=2
  Gain1 : Gain  Gain=k
  Gain2 : Gain  Gain=1e+4
  Product : Product
  Product1 : Product
  Subtract : Sum
  Subtract1 : Sum
  im : Outport
  wires:
  h/1 -> Gain/1
  Gain/1 -> Subtract/1
  q/1 -> Divide/2, Product1/1, Gain1/1
  Gain1/1 -> Product1/2
  Product1/1 -> Subtract/2
  eta/1 -> Gain2/1
  Gain2/1 -> Product/1
  um/1 -> Product/2
  Constant/1 -> Subtract1/1
  Product/1 -> Subtract1/2
  Divide/1 -> im/1
  Subtract/1 -> Divide/1
  Subtract1/1 -> Divide/3

== system structuri_avansate/ModelProces 2/Filtru ==
  q : Inport
  Integrator : Integrator  InitialCondition=q0
  Sum : Sum  Inputs=|+-
  q_f : Outport
  wires:
  Integrator/1 -> Sum/2, q_f/1
  q/1 -> Sum/1
  Sum/1 -> Integrator/1

== system structuri_avansate/ModelProces 2/Motor  ==
  um : Inport
  im : Inport  Port=2
  Add : Sum  Inputs=+-
  Rm : Gain  Gain=3
  kn : Outport
  wires:
  Rm/1 -> Add/2
  um/1 -> Add/1
  im/1 -> Rm/1
  Add/1 -> kn/1

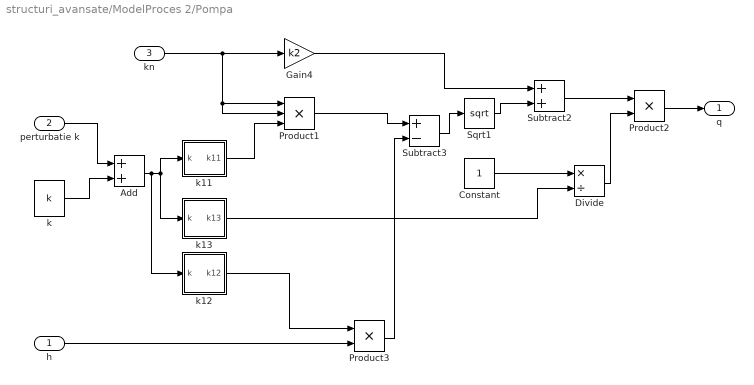
== system structuri_avansate/ModelProces 2/Pompa ==
  h : Inport
  perturbatie k : Inport  Port=2
  kn : Inport  Port=3
  Add : Sum
  Constant : Constant
  Divide : Product  Inputs=*/
  Gain4 : Gain  Gain=k2
  Product1 : Product  Inputs=3
  Product2 : Product
  Product3 : Product
  Sqrt1 : Sqrt
  Subtract2 : Sum
  Subtract3 : Sum  Inputs=+-
  "k " : Constant  Value=k
  "k11 " : Subsystem
  k12 : Subsystem
  k13 : Subsystem
  q : Outport
  wires:
  Product2/1 -> q/1
  Divide/1 -> Product2/2
  Sqrt1/1 -> Subtract2/2
  k13/1(k13) -> Divide/2
  Constant/1 -> Divide/1
  "k11 "/1(k11) -> Product1/3
  Product3/1 -> Subtract3/2
  k12/1(k12) -> Product3/1
  Subtract2/1 -> Product2/1
  Add/1 -> k12/1(k), k13/1(k), "k11 "/1(k)
  perturbatie k/1 -> Add/1
  "k "/1 -> Add/2
  Subtract3/1 -> Sqrt1/1
  kn/1 -> Product1/2, Product1/1, Gain4/1
  h/1 -> Product3/2
  Gain4/1 -> Subtract2/1
  Product1/1 -> Subtract3/1

== system structuri_avansate/ModelProces 2/Randament ==
  "q " : Inport
  um : Inport  Port=2
  Gain : Gain  Gain=8e-5
  Product : Product
  "eta " : Outport
  wires:
  um/1 -> Gain/1
  Gain/1 -> Product/2
  "q "/1 -> Product/1
  Product/1 -> "eta "/1

== system structuri_avansate/ModelProces 2/Rezervor ==
  q : Inport
  Gain : Gain  Gain=1/332.5
  Integrator : Integrator  InitialCondition=h0
  Product : Product
  Sqrt : Sqrt
  Sum : Sum  Inputs=|+-
  c : Constant  Value=C
  h : Outport
  wires:
  Sum/1 -> Gain/1
  Sqrt/1 -> Product/1
  q/1 -> Sum/1
  Gain/1 -> Integrator/1
  Product/1 -> Sum/2
  c/1 -> Product/2
  Integrator/1 -> h/1, Sqrt/1

== system structuri_avansate/ModelProces 3/Amplificator  ==
  ua : Inport
  Constant : Constant  Value=8.1
  Gain : Gain  Gain=2.2
  Gain1 : Gain  Gain=2.2
  Gain2 : Gain  Gain=5
  Saturation : Saturate  UpperLimit=22  LowerLimit=0
  Sum : Sum  Inputs=|++
  Sum1 : Sum  Inputs=|+-
  Switch : Switch  Threshold=8.1  SaturateOnIntegerOverflow=off  InputSameDT=off
  "um " : Outport
  wires:
  Sum1/1 -> Gain2/1
  ua/1 -> Switch/2, Gain/1, Sum1/1, Gain1/1
  Gain2/1 -> Sum/2
  Gain1/1 -> Sum/1
  Sum/1 -> Switch/1
  Gain/1 -> Switch/3
  Constant/1 -> Sum1/2
  Switch/1 -> Saturation/1
  Saturation/1 -> "um "/1

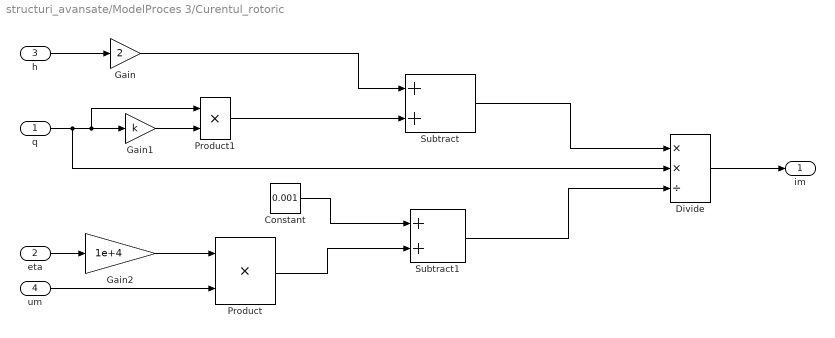
== system structuri_avansate/ModelProces 3/Curentul_rotoric ==
  q : Inport
  eta : Inport  Port=2
  h : Inport  Port=3
  um : Inport  Port=4
  Constant : Constant  Value=0.001
  Divide : Product  Inputs=**/
  Gain : Gain  Gain=2
  Gain1 : Gain  Gain=k
  Gain2 : Gain  Gain=1e+4
  Product : Product
  Product1 : Product
  Subtract : Sum
  Subtract1 : Sum
  im : Outport
  wires:
  h/1 -> Gain/1
  Gain/1 -> Subtract/1
  q/1 -> Divide/2, Product1/1, Gain1/1
  Gain1/1 -> Product1/2
  Product1/1 -> Subtract/2
  eta/1 -> Gain2/1
  Gain2/1 -> Product/1
  um/1 -> Product/2
  Constant/1 -> Subtract1/1
  Product/1 -> Subtract1/2
  Divide/1 -> im/1
  Subtract/1 -> Divide/1
  Subtract1/1 -> Divide/3

== system structuri_avansate/ModelProces 3/Filtru ==
  q : Inport
  Integrator : Integrator  InitialCondition=q0
  Sum : Sum  Inputs=|+-
  q_f : Outport
  wires:
  Integrator/1 -> Sum/2, q_f/1
  q/1 -> Sum/1
  Sum/1 -> Integrator/1

== system structuri_avansate/ModelProces 3/Motor  ==
  um : Inport
  im : Inport  Port=2
  Add : Sum  Inputs=+-
  Rm : Gain  Gain=3
  kn : Outport
  wires:
  Rm/1 -> Add/2
  um/1 -> Add/1
  im/1 -> Rm/1
  Add/1 -> kn/1

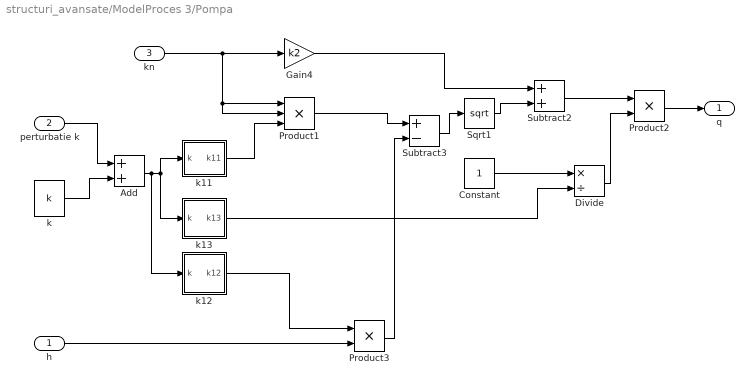
== system structuri_avansate/ModelProces 3/Pompa ==
  h : Inport
  perturbatie k : Inport  Port=2
  kn : Inport  Port=3
  Add : Sum
  Constant : Constant
  Divide : Product  Inputs=*/
  Gain4 : Gain  Gain=k2
  Product1 : Product  Inputs=3
  Product2 : Product
  Product3 : Product
  Sqrt1 : Sqrt
  Subtract2 : Sum
  Subtract3 : Sum  Inputs=+-
  "k " : Constant  Value=k
  "k11 " : Subsystem
  k12 : Subsystem
  k13 : Subsystem
  q : Outport
  wires:
  Product2/1 -> q/1
  Divide/1 -> Product2/2
  Sqrt1/1 -> Subtract2/2
  k13/1(k13) -> Divide/2
  Constant/1 -> Divide/1
  "k11 "/1(k11) -> Product1/3
  Product3/1 -> Subtract3/2
  k12/1(k12) -> Product3/1
  Subtract2/1 -> Product2/1
  Add/1 -> k12/1(k), k13/1(k), "k11 "/1(k)
  perturbatie k/1 -> Add/1
  "k "/1 -> Add/2
  Subtract3/1 -> Sqrt1/1
  kn/1 -> Product1/2, Product1/1, Gain4/1
  h/1 -> Product3/2
  Gain4/1 -> Subtract2/1
  Product1/1 -> Subtract3/1

== system structuri_avansate/ModelProces 3/Randament ==
  "q " : Inport
  um : Inport  Port=2
  Gain : Gain  Gain=8e-5
  Product : Product
  "eta " : Outport
  wires:
  um/1 -> Gain/1
  Gain/1 -> Product/2
  "q "/1 -> Product/1
  Product/1 -> "eta "/1

== system structuri_avansate/ModelProces 3/Rezervor ==
  q : Inport
  Gain : Gain  Gain=1/332.5
  Integrator : Integrator  InitialCondition=h0
  Product : Product
  Sqrt : Sqrt
  Sum : Sum  Inputs=|+-
  c : Constant  Value=C
  h : Outport
  wires:
  Sum/1 -> Gain/1
  Sqrt/1 -> Product/1
  q/1 -> Sum/1
  Gain/1 -> Integrator/1
  Product/1 -> Sum/2
  c/1 -> Product/2
  Integrator/1 -> h/1, Sqrt/1

== system structuri_avansate/ModelProces 4/Amplificator  ==
  ua : Inport
  Constant : Constant  Value=8.1
  Gain : Gain  Gain=2.2
  Gain1 : Gain  Gain=2.2
  Gain2 : Gain  Gain=5
  Saturation : Saturate  UpperLimit=22  LowerLimit=0
  Sum : Sum  Inputs=|++
  Sum1 : Sum  Inputs=|+-
  Switch : Switch  Threshold=8.1  SaturateOnIntegerOverflow=off  InputSameDT=off
  "um " : Outport
  wires:
  Sum1/1 -> Gain2/1
  ua/1 -> Switch/2, Gain/1, Sum1/1, Gain1/1
  Gain2/1 -> Sum/2
  Gain1/1 -> Sum/1
  Sum/1 -> Switch/1
  Gain/1 -> Switch/3
  Constant/1 -> Sum1/2
  Switch/1 -> Saturation/1
  Saturation/1 -> "um "/1

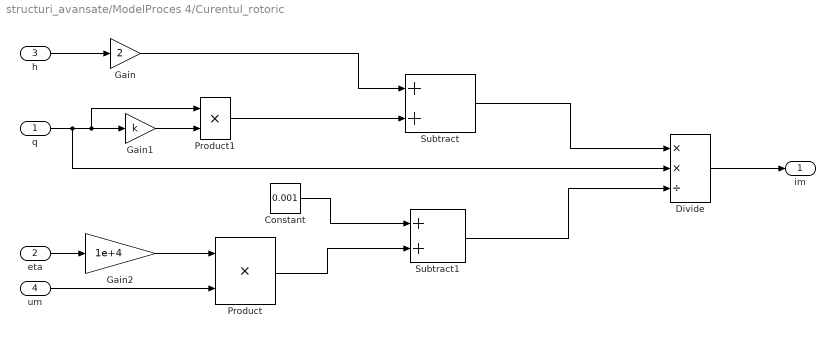
== system structuri_avansate/ModelProces 4/Curentul_rotoric ==
  q : Inport
  eta : Inport  Port=2
  h : Inport  Port=3
  um : Inport  Port=4
  Constant : Constant  Value=0.001
  Divide : Product  Inputs=**/
  Gain : Gain  Gain=2
  Gain1 : Gain  Gain=k
  Gain2 : Gain  Gain=1e+4
  Product : Product
  Product1 : Product
  Subtract : Sum
  Subtract1 : Sum
  im : Outport
  wires:
  h/1 -> Gain/1
  Gain/1 -> Subtract/1
  q/1 -> Divide/2, Product1/1, Gain1/1
  Gain1/1 -> Product1/2
  Product1/1 -> Subtract/2
  eta/1 -> Gain2/1
  Gain2/1 -> Product/1
  um/1 -> Product/2
  Constant/1 -> Subtract1/1
  Product/1 -> Subtract1/2
  Divide/1 -> im/1
  Subtract/1 -> Divide/1
  Subtract1/1 -> Divide/3

== system structuri_avansate/ModelProces 4/Filtru ==
  q : Inport
  Integrator : Integrator  InitialCondition=q0
  Sum : Sum  Inputs=|+-
  q_f : Outport
  wires:
  Integrator/1 -> Sum/2, q_f/1
  q/1 -> Sum/1
  Sum/1 -> Integrator/1

== system structuri_avansate/ModelProces 4/Motor  ==
  um : Inport
  im : Inport  Port=2
  Add : Sum  Inputs=+-
  Rm : Gain  Gain=3
  kn : Outport
  wires:
  Rm/1 -> Add/2
  um/1 -> Add/1
  im/1 -> Rm/1
  Add/1 -> kn/1

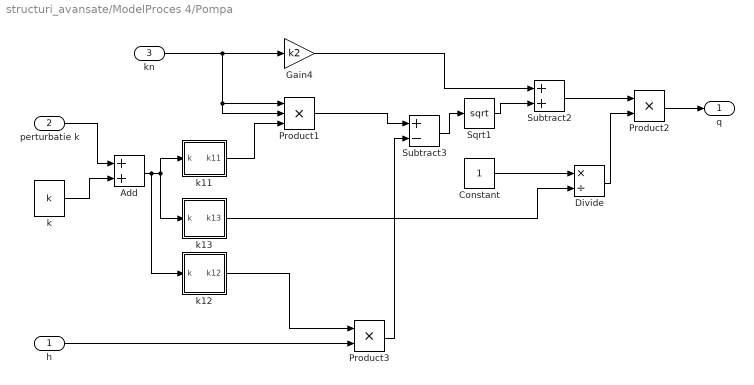
== system structuri_avansate/ModelProces 4/Pompa ==
  h : Inport
  perturbatie k : Inport  Port=2
  kn : Inport  Port=3
  Add : Sum
  Constant : Constant
  Divide : Product  Inputs=*/
  Gain4 : Gain  Gain=k2
  Product1 : Product  Inputs=3
  Product2 : Product
  Product3 : Product
  Sqrt1 : Sqrt
  Subtract2 : Sum
  Subtract3 : Sum  Inputs=+-
  "k " : Constant  Value=k
  "k11 " : Subsystem
  k12 : Subsystem
  k13 : Subsystem
  q : Outport
  wires:
  Product2/1 -> q/1
  Divide/1 -> Product2/2
  Sqrt1/1 -> Subtract2/2
  k13/1(k13) -> Divide/2
  Constant/1 -> Divide/1
  "k11 "/1(k11) -> Product1/3
  Product3/1 -> Subtract3/2
  k12/1(k12) -> Product3/1
  Subtract2/1 -> Product2/1
  Add/1 -> k12/1(k), k13/1(k), "k11 "/1(k)
  perturbatie k/1 -> Add/1
  "k "/1 -> Add/2
  Subtract3/1 -> Sqrt1/1
  kn/1 -> Product1/2, Product1/1, Gain4/1
  h/1 -> Product3/2
  Gain4/1 -> Subtract2/1
  Product1/1 -> Subtract3/1

== system structuri_avansate/ModelProces 4/Randament ==
  "q " : Inport
  um : Inport  Port=2
  Gain : Gain  Gain=8e-5
  Product : Product
  "eta " : Outport
  wires:
  um/1 -> Gain/1
  Gain/1 -> Product/2
  "q "/1 -> Product/1
  Product/1 -> "eta "/1

== system structuri_avansate/ModelProces 4/Rezervor ==
  q : Inport
  Add : Sum
  Constant : Constant  Value=C
  Gain : Gain  Gain=1/332.5
  Integrator : Integrator  InitialCondition=h0
  Product : Product
  Product1 : Product
  Scope : Scope
  Sqrt : Sqrt
  Step : Step  Time=500  After=4  SampleTime=0
  Sum : Sum  Inputs=|+-
  h : Outport
  perturbatie : Outport  Port=2
  wires:
  Step/1 -> Product1/2, Add/1
  Sqrt/1 -> Product1/1, Product/1
  Gain/1 -> Integrator/1
  Add/1 -> Product/2
  Constant/1 -> Add/2
  q/1 -> Sum/1
  Sum/1 -> Gain/1
  Product/1 -> Scope/1, Sum/2
  Product1/1 -> perturbatie/1
  Integrator/1 -> Sqrt/1, h/1

== system structuri_avansate/ModelProces 1/Pompa/k11  ==
  k : Inport
  Add : Sum
  Constant : Constant  Value=4
  Product : Product
  Product1 : Product  Inputs=3
  Subtract : Sum  Inputs=+-
  k1 : Constant  Value=0.624
  k2 : Constant  Value=-0.015
  k3 : Constant  Value=-0.0006
  k11 : Outport
  wires:
  k2/1 -> Product/2, Product/1
  k/1 -> Subtract/1
  k3/1 -> Subtract/2
  Subtract/1 -> Product1/1
  k1/1 -> Product1/2
  Constant/1 -> Product1/3
  Product1/1 -> Add/1
  Product/1 -> Add/2
  Add/1 -> k11/1

== system structuri_avansate/ModelProces 1/Pompa/k12 ==
  k : Inport
  Product1 : Product
  Subtract : Sum  Inputs=+-
  "constant " : Constant  Value=8
  k3 : Constant  Value=-0.0006
  k12 : Outport
  wires:
  k/1 -> Subtract/1
  k3/1 -> Subtract/2
  Subtract/1 -> Product1/1
  "constant "/1 -> Product1/2
  Product1/1 -> k12/1

== system structuri_avansate/ModelProces 1/Pompa/k13 ==
  k : Inport
  Product1 : Product
  Subtract : Sum  Inputs=+-
  "constant " : Constant  Value=2
  k3 : Constant  Value=-0.0006
  k13 : Outport
  wires:
  k/1 -> Subtract/1
  k3/1 -> Subtract/2
  Subtract/1 -> Product1/1
  "constant "/1 -> Product1/2
  Product1/1 -> k13/1

== system structuri_avansate/ModelProces 2/Pompa/k11  ==
  k : Inport
  Add : Sum
  Constant : Constant  Value=4
  Product : Product
  Product1 : Product  Inputs=3
  Subtract : Sum  Inputs=+-
  k1 : Constant  Value=0.624
  k2 : Constant  Value=-0.015
  k3 : Constant  Value=-0.0006
  k11 : Outport
  wires:
  k2/1 -> Product/2, Product/1
  k/1 -> Subtract/1
  k3/1 -> Subtract/2
  Subtract/1 -> Product1/1
  k1/1 -> Product1/2
  Constant/1 -> Product1/3
  Product1/1 -> Add/1
  Product/1 -> Add/2
  Add/1 -> k11/1

== system structuri_avansate/ModelProces 2/Pompa/k12 ==
  k : Inport
  Product1 : Product
  Subtract : Sum  Inputs=+-
  "constant " : Constant  Value=8
  k3 : Constant  Value=-0.0006
  k12 : Outport
  wires:
  k/1 -> Subtract/1
  k3/1 -> Subtract/2
  Subtract/1 -> Product1/1
  "constant "/1 -> Product1/2
  Product1/1 -> k12/1

== system structuri_avansate/ModelProces 2/Pompa/k13 ==
  k : Inport
  Product1 : Product
  Subtract : Sum  Inputs=+-
  "constant " : Constant  Value=2
  k3 : Constant  Value=-0.0006
  k13 : Outport
  wires:
  k/1 -> Subtract/1
  k3/1 -> Subtract/2
  Subtract/1 -> Product1/1
  "constant "/1 -> Product1/2
  Product1/1 -> k13/1
